simulink model "Control_OnOff_y_OnOff_con_histeresis"  (R2024b)
settings: Solver=VariableStepAuto  StartTime=0.0  StopTime=20  RelTol=1e-3
settings Model: Creator=geova  LastModifiedBy=geova

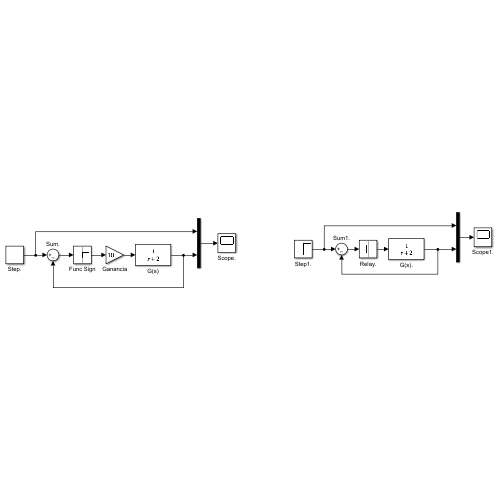
[thumbnail: Simulink's stored preview of the top-level diagram]
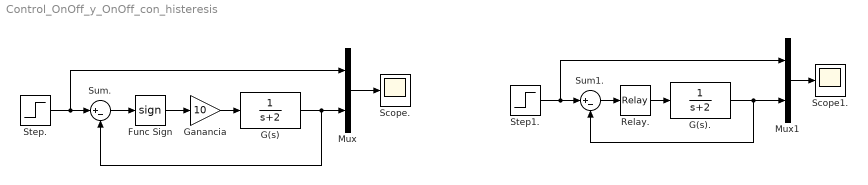
== system Control_OnOff_y_OnOff_con_histeresis ==
  Func Sign : Signum  ZeroCross=off
  G(s) : TransferFcn  Denominator=[1 2]
  G(s). : TransferFcn  Denominator=[1 2]
  Ganancia : Gain  Gain=10
  Mux : Mux  Inputs=2
  Mux1 : Mux  Inputs=2
  Relay. : Relay  OnSwitchValue=0.05  OffSwitchValue=-0.05  OnOutputValue=10  OffOutputValue=2
  Scope. : Scope
  Scope1. : Scope
  Step. : Step  Time=10  Before=1  After=2  SampleTime=0
  Step1. : Step  Time=10  Before=1  After=2  SampleTime=0
  Sum. : Sum  Inputs=|+-
  Sum1. : Sum  Inputs=|+-
  wires:
  Func Sign/1 -> Ganancia/1
  G(s)/1 -> Mux/2, Sum./2
  Step./1 -> Mux/1, Sum./1
  Sum./1 -> Func Sign/1
  Mux/1 -> Scope./1
  Ganancia/1 -> G(s)/1
  Relay./1 -> G(s)./1
  Sum1./1 -> Relay./1
  G(s)./1 -> Mux1/2, Sum1./2
  Step1./1 -> Mux1/1, Sum1./1
  Mux1/1 -> Scope1./1
